simulink model "FCS_flight_Fixed_Wing"  (R2025a)
settings: Solver=ode3  StartTime=0.0  StopTime=inf  FixedStep=FC.samp_time  MaxStep=1e-2  RelTol=1e-3  AbsTol=1e-3  EnableMultiTasking=on
libraries: simulink x1
settings Model: ExtModeTrigDuration=10  Creator=gurt1  LastModifiedBy=gurt1
settings SolverCC: PositivePriorityOrder=on
settings OptimizationCC: EnhancedBackFolding=on  PassReuseOutputArgsAs=Individual arguments  ZeroExternalMemoryAtStartup=off  ZeroInternalMemoryAtStartup=off  MaxStackSize=64  OptimizeBlockOrder=speed  DifferentSizesBufferReuse=on  OptimizationCustomize=off  EfficientTunableParamExpr=on
settings DebuggingCC: ParameterTunabilityLossMsg=error
settings HardwareCC: ProdBitPerPointer=32.0  ProdBitPerSizeT=32.0  ProdBitPerPtrDiffT=32.0  ProdLargestAtomicInteger=Long  ProdLargestAtomicFloat=Double  ProdWordSize=32.0  ProdLongLongMode=on  ProdHWDeviceType=ARM Compatible->ARM Cortex
settings SFSimCC: MATLABDynamicMemAlloc=off  SimTargetLang=C++  SimDLTargetLibrary=mkl-dnn
settings RTWCC: SystemTargetFile=ert.tlc  HardwareBoard=PX4 Cube Orange  TLCOptions="-aInlineSetEventsForThisBaseRateFcn=TLC_FALSE -aSuppressMultiTaskScheduler=TLC_FALSE  -aRateBasedStepFcn=0"  TemplateMakefile=ert_default_tmf  Toolchain=GNU Tools for PX4 Autopilots  TargetLang=C++  GPUComputeCapability=3.5  Description=Embedded Coder
settings CodeAppCC: ForceParamTrailComments=on  IgnoreCustomStorageClasses=off  OperatorAnnotations=on  SimulinkDataObjDesc=on  SFDataObjDesc=on  InsertBlockDesc=on
settings ERTTargetCC: ExtModeTransport=3.0  ExtModeStaticAllocSize=1024.0  InlinedParameterPlacement=Hierarchical  DynamicArrayContainerType=coder::array  SupportVariableSizeSignals=on

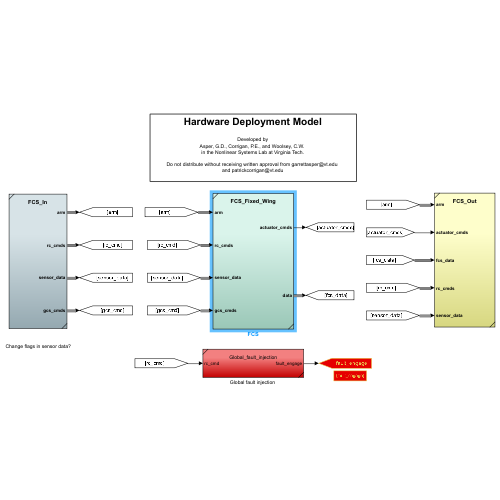
[thumbnail: Simulink's stored preview of the top-level diagram]
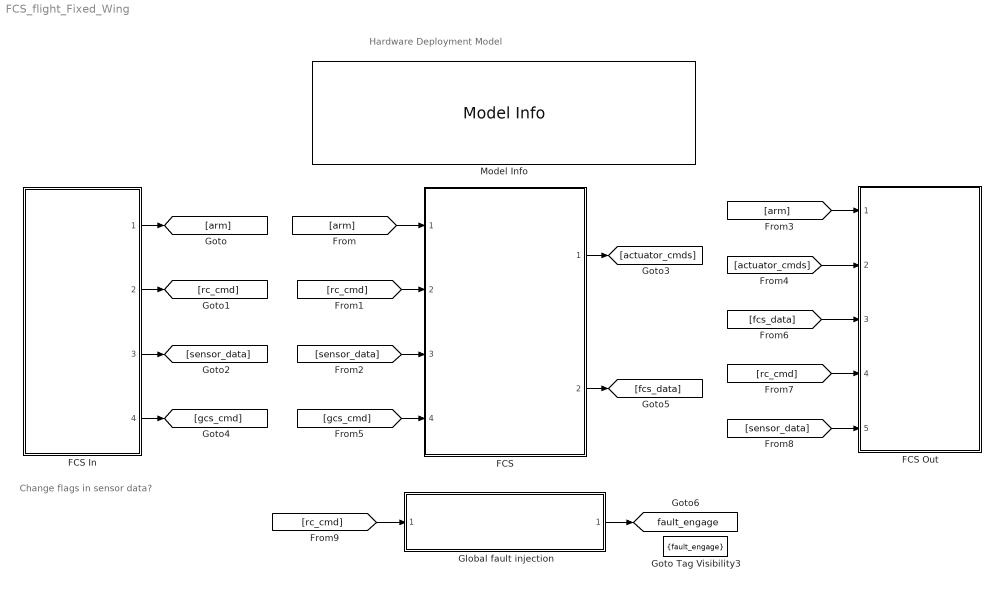
== system FCS_flight_Fixed_Wing ==
  note: Change flags in sensor data?
  note: Hardware Deployment Model
  FCS : Subsystem  ReferencedSubsystem=FCS_Fixed_Wing
  FCS In : Subsystem  ReferencedSubsystem=FCS_In
  FCS Out : Subsystem  ReferencedSubsystem=FCS_Out
  "Global fault injection " : Subsystem  ReferencedSubsystem=Global_fault_injection
  Goto Tag Visibility3 : GotoTagVisibility  GotoTag=fault_engage
  Model Info : simulink/Model-Wide Utilities/Model Info  Frame=off  DisplayStringWithTags=|  HorizontalTextAlignment=Center  LeftAlignmentValue=0.5
      | Developed by
      | Asper, G.D., Corrigan, P.E., and Woolsey, C.W. 
      | in the Nonlinear Systems Lab at Virginia Tech.
      | 
      | Do not distribute without receiving written approval from garrettasper@vt.edu 
      | and patrickcorrigan@vt.edu
  tag scope: fault_engage=global
  wires:
  [arm] -> FCS/1
  [rc_cmd] -> FCS/2
  [sensor_data] -> FCS/3
  FCS/1 -> [actuator_cmds]
  [gcs_cmd] -> FCS/4
  FCS/2 -> [fcs_data]
  FCS In/1 -> [arm]
  FCS In/2 -> [rc_cmd]
  FCS In/3 -> [sensor_data]
  FCS In/4 -> [gcs_cmd]
  [arm] -> FCS Out/1
  [actuator_cmds] -> FCS Out/2
  [fcs_data] -> FCS Out/3
  [rc_cmd] -> FCS Out/4
  [sensor_data] -> FCS Out/5
  [rc_cmd] -> "Global fault injection "/1
  "Global fault injection "/1 -> [fault_engage]
